simulink model "LSTM_sim"  (R2018a)
settings: Solver=VariableStepAuto  StartTime=0.0  StopTime=10.0  RelTol=1e-3
undefined symbols (not defined in the file): b, Default_Output, FullyConnected_Bias, FullyConnected_Weights, Last_result, R, W, WormUp_Time
libraries: neural x4
settings Model: Creator=Hyunki  LastModifiedBy=Hyunki

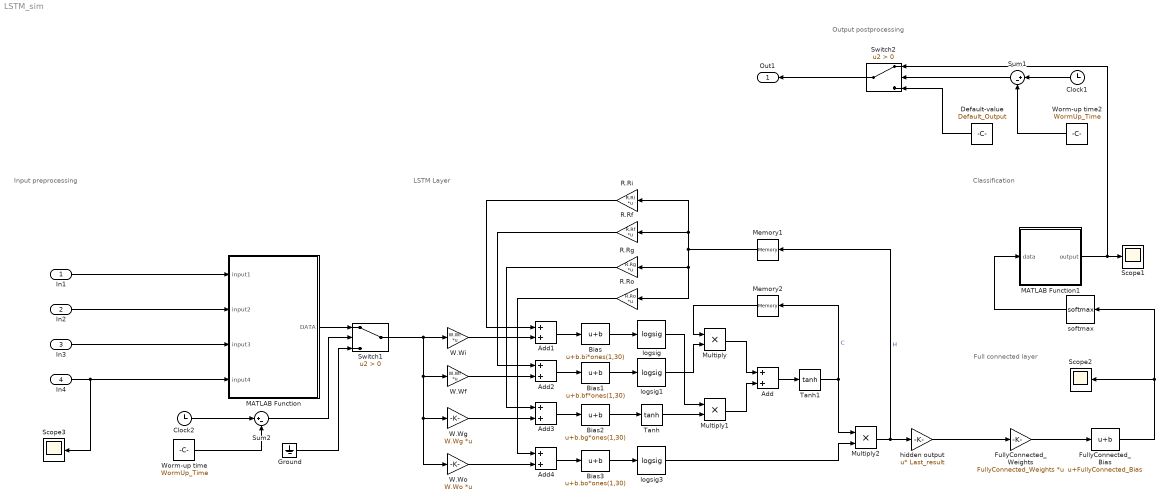
== system LSTM_sim ==
  note: Output postprocessing
  note: Classification
  note: Input preprocessing
  note: LSTM Layer
  note: Full connected layer
  In1 : Inport
  In2 : Inport  Port=2
  In3 : Inport  Port=3
  In4 : Inport  Port=4
  Add{,1..4} (5 alike) : Sum
  Bias : Bias  Bias=b.bi*ones(1,30)
  Bias1 : Bias  Bias=b.bf*ones(1,30)
  Bias2 : Bias  Bias=b.bg*ones(1,30)
  Bias3 : Bias  Bias=b.bo*ones(1,30)
  Clock1 : Clock
  Clock2 : Clock
  Default-value : Constant  Value=Default_Output
  FullyConnected_Bias : Bias  Bias=FullyConnected_Bias
  FullyConnected_Weights : Gain  Gain=FullyConnected_Weights  Multiplication=Matrix(K*u)
  Ground : Ground
  MATLAB Function : MATLAB Function  TreatAsAtomicUnit=on
  MATLAB Function1 : MATLAB Function  TreatAsAtomicUnit=on
  Memory1 : Memory
  Memory2 : Memory
  Multiply : Product
  Multiply1 : Product
  Multiply2 : Product
  R.Rf : Gain  Gain=R.Rf  Multiplication=Matrix(K*u)
  R.Rg : Gain  Gain=R.Rg  Multiplication=Matrix(K*u)
  R.Ri : Gain  Gain=R.Ri  Multiplication=Matrix(K*u)
  R.Ro : Gain  Gain=R.Ro  Multiplication=Matrix(K*u)
  Scope1 : Scope
  Scope2 : Scope
  Scope3 : Scope
  Sum1 : Sum  Inputs=|+-
  Sum2 : Sum  Inputs=|+-
  Switch1 : Switch  Criteria=u2 > Threshold
  Switch2 : Switch  Criteria=u2 > Threshold
  Tanh : Trigonometry  Operator=tanh
  Tanh1 : Trigonometry  Operator=tanh
  W.Wf : Gain  Gain=W.Wf  Multiplication=Matrix(K*u)
  W.Wg : Gain  Gain=W.Wg  Multiplication=Matrix(K*u)
  W.Wi : Gain  Gain=W.Wi  Multiplication=Matrix(K*u)
  W.Wo : Gain  Gain=W.Wo  Multiplication=Matrix(K*u)
  Worm-up time : Constant  Value=WormUp_Time
  Worm-up time2 : Constant  Value=WormUp_Time
  hidden output : Gain  Gain=Last_result  Multiplication=Matrix(u*K)
  logsig : neural/Transfer Functions/logsig
      settings: SourceProductName=Neural Network Toolbox  SourceProductBaseCode=NN
  logsig1 : neural/Transfer Functions/logsig
      settings: SourceProductName=Neural Network Toolbox  SourceProductBaseCode=NN
  logsig3 : neural/Transfer Functions/logsig
      settings: SourceProductName=Neural Network Toolbox  SourceProductBaseCode=NN
  softmax : neural/Transfer Functions/softmax
      settings: SourceProductName=Neural Network Toolbox  SourceProductBaseCode=NN
  Out1 : Outport
  wires:
  MATLAB Function/1(DATA) -> Switch1/1
  Memory1/1 -> R.Ro/1, R.Rg/1, R.Ri/1, R.Rf/1
  Bias2/1 -> Tanh/1
  Bias3/1 -> logsig3/1
  Tanh1/1 -> Multiply2/1, Memory2/1  "C"
  In4/1 -> MATLAB Function/4(input4), Scope3/1
  logsig3/1 -> Multiply2/2
  R.Rf/1 -> Add2/1
  R.Ro/1 -> Add4/1
  In2/1 -> MATLAB Function/2(input2)
  FullyConnected_Bias/1 -> softmax/1, Scope2/1
  hidden output/1 -> FullyConnected_Weights/1
  Clock1/1 -> Sum1/1
  Switch2/1 -> Out1/1
  Tanh/1 -> Multiply1/2
  Ground/1 -> Switch1/3
  Bias1/1 -> logsig1/1
  In1/1 -> MATLAB Function/1(input1)
  Worm-up time/1 -> Sum2/2
  Sum1/1 -> Switch2/2
  Multiply/1 -> Add/1
  Sum2/1 -> Switch1/2
  Memory2/1 -> Multiply/1
  logsig/1 -> Multiply1/1
  Add3/1 -> Bias2/1
  Multiply1/1 -> Add/2
  Worm-up time2/1 -> Sum1/2
  Add2/1 -> Bias1/1
  Add4/1 -> Bias3/1
  Clock2/1 -> Sum2/1
  Add1/1 -> Bias/1
  logsig1/1 -> Multiply/2
  Default-value/1 -> Switch2/3
  FullyConnected_Weights/1 -> FullyConnected_Bias/1
  R.Ri/1 -> Add1/1
  In3/1 -> MATLAB Function/3(input3)
  R.Rg/1 -> Add3/1
  W.Wo/1 -> Add4/2
  W.Wi/1 -> Add1/2
  W.Wg/1 -> Add3/2
  softmax/1 -> MATLAB Function1/1(data)
  Multiply2/1 -> hidden output/1, Memory1/1  "H"
  W.Wf/1 -> Add2/2
  Switch1/1 -> W.Wf/1, W.Wg/1, W.Wo/1, W.Wi/1
  MATLAB Function1/1(output) -> Scope1/1, Switch2/1
  Add/1 -> Tanh1/1
  Bias/1 -> logsig/1

== matlab function LSTM_sim/MATLAB Function1 ==
  data: data input; output output
function output = categorize(data)

[~,index] = max(data(:,end));

if index == 1
    class = 1;
elseif index == 2
    class = 2;
elseif index == 2
    class = 2;
elseif index == 3
    class = 3;
elseif index == 4
    class = 4;
elseif index == 5
    class = 5;
else
    class = 6;
end
    
output = class;

== matlab function LSTM_sim/MATLAB Function ==
  data: DATA output; input1 input; input2 input; input3 input; input4 input
function DATA = Data_stack(input1,input2,input3,input4)

persistent save_input1; 
persistent save_input2; 
persistent save_input3; 
persistent save_input4; 

if isempty(save_input1)
    save_input1 = zeros(1,SequenceLength);
    save_input2 = zeros(1,SequenceLength);
    save_input3 = zeros(1,SequenceLength);
    save_input4 = zeros(1,SequenceLength);
end

for i = SequenceLength:-1:2
    save_input1(i) = save_input1(i-1);
    save_input2(i) = save_input2(i-1);
    save_input3(i) = save_input3(i-1);
    save_input4(i) = save_input4(i-1);
end

save_input1(1) = input1;
save_input2(1) = input2;
save_input3(1) = input3;
save_input4(1) = input4;


DATA = [save_input1;save_input2;save_input3;save_input4];
